simulink library "uas_pilot_model_r6"  (R2018b)
settings: Solver=VariableStepAuto  StartTime=0.0  StopTime=10.0  RelTol=1e-3
values from neighbouring files (symbols this model uses):
  deterministicMode = false    [HeuristicOperatorModelR6.m]
undefined symbols (not defined in the file or in its folder): alt_k, alt_offset, alt_theta, coord_delay_k, coord_delay_min, coord_delay_theta, dt, max_hdg_diff, mean_exec_delay, mean_initial_delay, mean_upd_times, min_exec_delay, min_initial_delay, min_upd_times, operator_enabled, prob_descend, prob_follow_min, prob_turn, prob_turn_left, rng_seed_coord, rng_seed_execution, rng_seed_horz, rng_seed_horz_vs_vert, rng_seed_initial, rng_seed_update, rng_seed_vert, turn_k, turn_k_alt, turn_offset, turn_offset_alt, turn_theta, turn_theta_alt
libraries: simulink x10
(part 1 of 2)
settings Model: Creator=RA24876  LastModifiedBy=PE29732
settings SFSimCC: SimUseLocalCustomCode=off
settings RTWCC: RTWUseLocalCustomCode=off
settings CodeAppCC: StateflowObjectComments=on

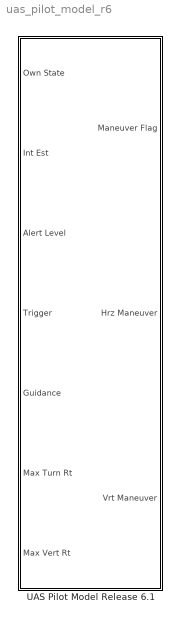
== system uas_pilot_model_r6 ==
  UAS Pilot Model Release 6.1 : Subsystem  TreatAsAtomicUnit=on  mask{dt=dt, operator_enabled=operator_enabled, deterministicMode=deterministicMode, mean_initial_delay=mean_initial_delay, min_initial_delay=min_initial_delay, coord_delay_k=coord_delay_k, coord_delay_theta=coord_delay_theta, coord_delay_min=coord_delay_min, mean_exec_delay=mean_exec_delay, min_exec_delay=min_exec_delay, min_upd_times=min_upd_times, mean_upd_times=mean_upd_times, rng_seed_initial=rng_seed_initial, rng_seed_coord=rng_seed_coord, rng_seed_execution=rng_seed_execution, rng_seed_update=rng_seed_update, prob_follow_min=prob_follow_min, prob_turn_left=prob_turn_left, prob_turn_table=prob_turn, max_hdg_diff=max_hdg_diff, prob_descend=prob_descend, turn_k=turn_k, turn_theta=turn_theta, turn_offset=turn_offset, turn_k_alt=turn_k_alt, turn_theta_alt=turn_theta_alt, turn_offset_alt=turn_offset_alt, alt_k=alt_k, alt_theta=alt_theta, alt_offset=alt_offset, rng_seed_horz=rng_seed_horz, rng_seed_vert=rng_seed_vert, rng_seed_horz_vs_vert=rng_seed_horz_vs_vert, mental_filter_samples=0, mental_filter_climb_thresh=0, mental_filter_turn_thresh=0}
      mask prompts: dt "Sample Time (s)"; operator_enabled "Enable Pilot Model (T/F)"; deterministicMode "Deterministic Mode"; mean_initial_delay "Mean Initial Delay (s)"; min_initial_delay "Minimum Initial Delay (s)"; coord_delay_k "Coordination Delay Gamma Distribution Shape Parameter, k"; coord_delay_theta "Coordination Delay Gamma Distribuition Scale Parameter, theta"; coord_delay_min "Minimum Coordination Delay (s)"; mean_exec_delay "Mean Execution Delay (s)"; min_exec_delay "Minimum Execution Delay (s)"; min_upd_times "Minimum Maneuve Update Times by Alert Level (s)"; mean_upd_times "Mean Maneuver Update Time by Alert Level (s)"; rng_seed_initial "Random Seed (Initial Delay)"; rng_seed_coord "Random Seed (Coord Delay)"; rng_seed_execution "Random Seed (Exec Delay)"; rng_seed_update "Random Seed (Update Delay)"; prob_follow_min "Probability of Following Minimum Guidance"; prob_turn_left "Probability of Turning Left"; prob_turn_table "Probability of Choosing Turn"; max_hdg_diff "Maximum Heading Difference to Override (deg)"; prob_descend "Probability of Descend vs. Climb"; turn_k "Primary Turn Magnitude Gamma Distribution Shape Parameter"; turn_theta "Primary Turn Magnitude Gamma Distribution Scale Parameter"; turn_offset "Primary Turn Magnitude Offset (deg)"; turn_k_alt "Alternate Turn Magnitude Shape Parameter"; turn_theta_alt "Alternate Turn Magnitude Scale Parameter"; turn_offset_alt "Alternate Turn Magnitude Offset"; alt_k "Altitude Gamma Distribution Shape Parameter"; alt_theta "Altitude Gamma Distribution Scale Parameter"; alt_offset "Altitude Offset (ft)"; rng_seed_horz "Random Seed (Horz Maneuver)"; rng_seed_vert "Random Seed (Vert Maneuver)"; rng_seed_horz_vs_vert "Random Seed (Turn vs. Climb)"; mental_filter_samples "Number of Samples for Mental Filter"; mental_filter_climb_thresh "Mental Filter Climb Threshold (fps)"; mental_filter_turn_thresh "Mental Filter Turn Threshold (rad)"
      mask DialogControl DescGroupVar Prompt: UAS Pilot Model
      mask DialogControl DescTextVar Prompt: Response of UAS pilot to intruder causing a DAA alert

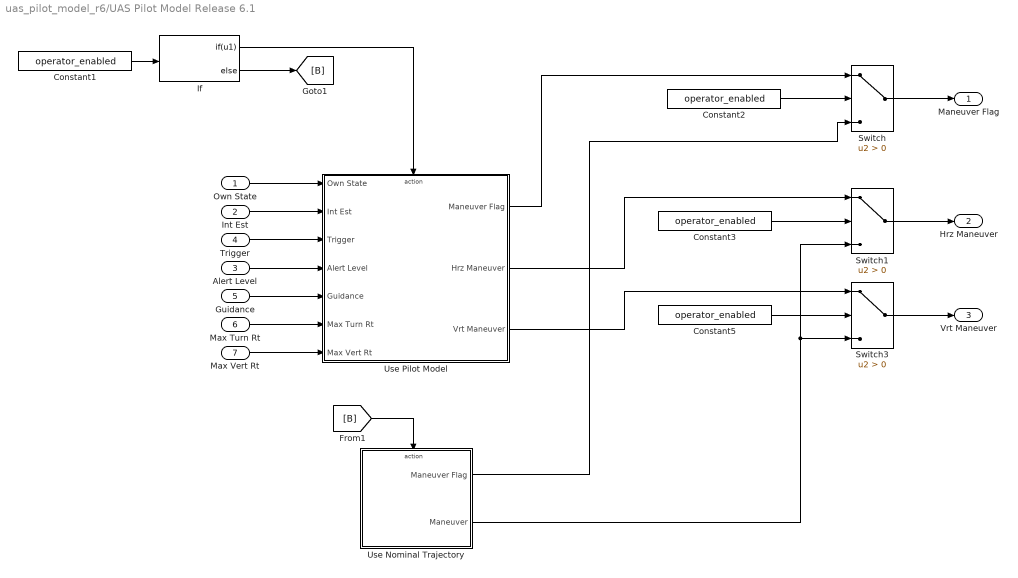
== system uas_pilot_model_r6/UAS Pilot Model Release 6.1 ==
  Own State : Inport  OutDataTypeStr=Bus: AircraftState
  Int Est : Inport  Port=2  OutDataTypeStr=Bus: AircraftEstimate
  Alert Level : Inport  Port=3
  Trigger : Inport  Port=4
  Guidance : Inport  Port=5
  Max Turn Rt : Inport  Port=6
  Max Vert Rt : Inport  Port=7
  Constant{1..3,5} (4 alike) : Constant  Value=operator_enabled  SampleTime=1
  If : If  IfExpression=u1
  Switch : Switch  Criteria=u2 > Threshold
  Switch1 : Switch  Criteria=u2 > Threshold
  Switch3 : Switch  Criteria=u2 > Threshold
  Use Nominal Trajectory : Subsystem  TreatAsAtomicUnit=on
  Use Pilot Model : Subsystem
  Maneuver Flag : Outport  OutDataTypeStr=boolean
  Hrz Maneuver : Outport  Port=2
  Vrt Maneuver : Outport  Port=3
  wires:
  Constant1/1 -> If/1
  If/2 -> [B]
  [B] -> Use Nominal Trajectory/Action
  Own State/1 -> Use Pilot Model/1(Own State)
  Int Est/1 -> Use Pilot Model/2(Int Est)
  If/1 -> Use Pilot Model/Action
  Switch/1 -> Maneuver Flag/1
  Constant2/1 -> Switch/2
  Use Pilot Model/1(Maneuver Flag) -> Switch/1
  Constant3/1 -> Switch1/2
  Use Pilot Model/2(Hrz Maneuver) -> Switch1/1
  Use Nominal Trajectory/1(Maneuver Flag) -> Switch/3
  Guidance/1 -> Use Pilot Model/5(Guidance)
  Constant5/1 -> Switch3/2
  Use Pilot Model/3(Vrt Maneuver) -> Switch3/1
  Use Nominal Trajectory/2(Maneuver) -> Switch3/3, Switch1/3
  Switch1/1 -> Hrz Maneuver/1
  Switch3/1 -> Vrt Maneuver/1
  Trigger/1 -> Use Pilot Model/3(Trigger)
  Alert Level/1 -> Use Pilot Model/4(Alert Level)
  Max Turn Rt/1 -> Use Pilot Model/6(Max Turn Rt)
  Max Vert Rt/1 -> Use Pilot Model/7(Max Vert Rt)

== system uas_pilot_model_r6/UAS Pilot Model Release 6.1/Use Nominal Trajectory ==
  Action Port : ActionPort
  Constant : Constant  Value=false
  Null Maneuver : Subsystem
  Maneuver Flag : Outport  InitialOutput=0
  Maneuver : Outport  Port=2  InitialOutput=0
  wires:
  Null Maneuver/1(Null) -> Maneuver/1
  Constant/1 -> Maneuver Flag/1

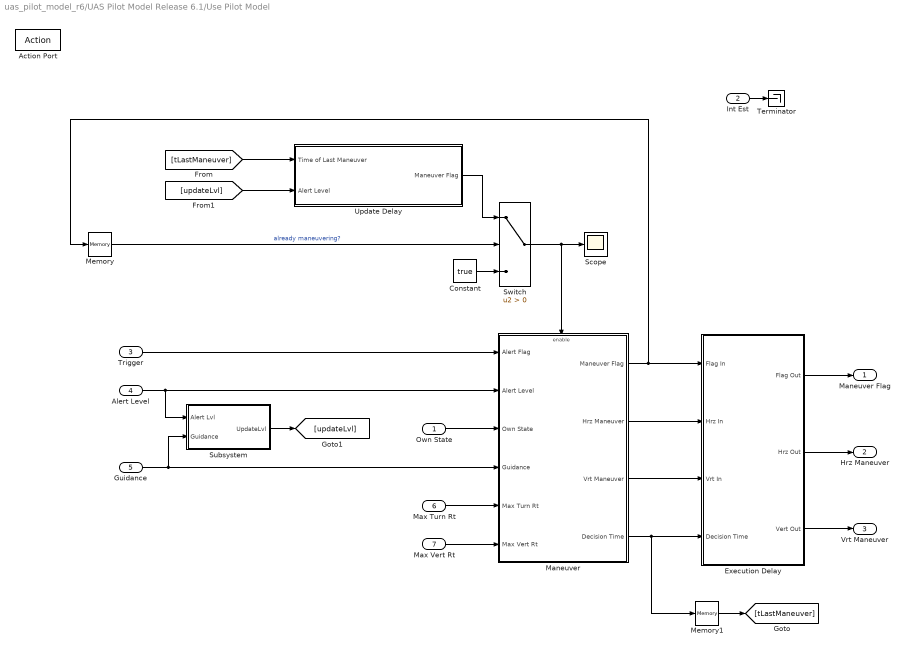
== system uas_pilot_model_r6/UAS Pilot Model Release 6.1/Use Pilot Model ==
  Own State : Inport  OutDataTypeStr=Bus: AircraftState
  Int Est : Inport  Port=2  OutDataTypeStr=Bus: AircraftEstimate
  Trigger : Inport  Port=3
  Alert Level : Inport  Port=4
  Guidance : Inport  Port=5
  Max Turn Rt : Inport  Port=6
  Max Vert Rt : Inport  Port=7
  Action Port : ActionPort
  Constant : Constant  Value=true
  Execution Delay : Subsystem
  Maneuver : Subsystem
  Memory : Memory  InheritSampleTime=on
  Memory1 : Memory  InheritSampleTime=on
  Scope : Scope
  Subsystem : Subsystem
  Switch : Switch  Criteria=u2 > Threshold
  Terminator : Terminator
  Update Delay : Subsystem
  Maneuver Flag : Outport  OutDataTypeStr=boolean
  Hrz Maneuver : Outport  Port=2
  Vrt Maneuver : Outport  Port=3
  wires:
  Maneuver/1(Maneuver Flag) -> Execution Delay/1(Flag In), Memory/1
  Guidance/1 -> Subsystem/2(Guidance), Maneuver/4(Guidance)
  Int Est/1 -> Terminator/1
  Constant/1 -> Switch/3
  Memory/1 -> Switch/2  "already maneuvering?"
  Own State/1 -> Maneuver/3(Own State)
  Trigger/1 -> Maneuver/1(Alert Flag)
  Alert Level/1 -> Subsystem/1(Alert Lvl), Maneuver/2(Alert Level)
  Switch/1 -> Maneuver/Enable, Scope/1
  Maneuver/2(Hrz Maneuver) -> Execution Delay/2(Hrz In)
  Maneuver/3(Vrt Maneuver) -> Execution Delay/3(Vrt In)
  Update Delay/1(Maneuver Flag) -> Switch/1
  Maneuver/4(Decision Time) -> Memory1/1, Execution Delay/4(Decision Time)
  Memory1/1 -> [tLastManeuver]
  [tLastManeuver] -> Update Delay/1(Time of Last Maneuver)
  Subsystem/1(UpdateLvl) -> [updateLvl]
  [updateLvl] -> Update Delay/2(Alert Level)
  Max Turn Rt/1 -> Maneuver/5(Max Turn Rt)
  Max Vert Rt/1 -> Maneuver/6(Max Vert Rt)
  Execution Delay/1(Flag Out) -> Maneuver Flag/1
  Execution Delay/2(Hrz Out) -> Hrz Maneuver/1
  Execution Delay/3(Vert Out) -> Vrt Maneuver/1

== system uas_pilot_model_r6/UAS Pilot Model Release 6.1/Use Nominal Trajectory/Null Maneuver ==
  Bus Creator : BusCreator  Inputs=5  OutDataTypeStr=Bus: AvoidanceManeuver
  Constant{,1..3} (4 alike) : Constant  Value=0
  Digital Clock : DigitalClock  SampleTime=dt
  Null : Outport
  wires:
  Constant2/1 -> Bus Creator/5  "wc_flag"
  Constant/1 -> Bus Creator/2  "type"
  Constant1/1 -> Bus Creator/3  "desired_state"
  Digital Clock/1 -> Bus Creator/1  "time"
  Bus Creator/1 -> Null/1
  Constant3/1 -> Bus Creator/4  "reference_state"

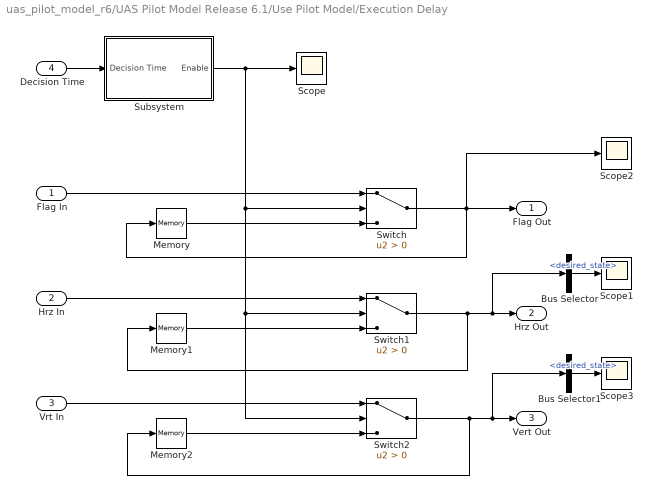
== system uas_pilot_model_r6/UAS Pilot Model Release 6.1/Use Pilot Model/Execution Delay ==
  Flag In : Inport
  Hrz In : Inport  Port=2
  Vrt In : Inport  Port=3
  Decision Time : Inport  Port=4
  Bus Selector : BusSelector  OutputSignals=desired_state
  Bus Selector1 : BusSelector  OutputSignals=desired_state
  Memory : Memory  InheritSampleTime=on
  Memory1 : Memory  InheritSampleTime=on
  Memory2 : Memory  InheritSampleTime=on
  Scope{,1..3} (4 alike) : Scope
  Subsystem : Subsystem
  Switch : Switch  Criteria=u2 > Threshold
  Switch1 : Switch  Criteria=u2 > Threshold
  Switch2 : Switch  Criteria=u2 > Threshold
  Flag Out : Outport
  Hrz Out : Outport  Port=2
  Vert Out : Outport  Port=3
  wires:
  Switch/1 -> Scope2/1, Memory/1, Flag Out/1
  Switch1/1 -> Memory1/1, Bus Selector/1, Hrz Out/1
  Flag In/1 -> Switch/1
  Vrt In/1 -> Switch2/1
  Hrz In/1 -> Switch1/1
  Memory/1 -> Switch/3
  Memory1/1 -> Switch1/3
  Memory2/1 -> Switch2/3
  Subsystem/1(Enable) -> Scope/1, Switch/2, Switch1/2, Switch2/2
  Decision Time/1 -> Subsystem/1(Decision Time)
  Bus Selector/1 -> Scope1/1  "<desired_state>"
  Switch2/1 -> Memory2/1, Bus Selector1/1, Vert Out/1
  Bus Selector1/1 -> Scope3/1  "<desired_state>"

== system uas_pilot_model_r6/UAS Pilot Model Release 6.1/Use Pilot Model/Maneuver ==
  Alert Flag : Inport
  Alert Level : Inport  Port=2
  Own State : Inport  Port=3
  Guidance : Inport  Port=4
  Max Turn Rt : Inport  Port=5
  Max Vert Rt : Inport  Port=6
  Enable : EnablePort
  Coordination Delay : Subsystem
  Initial Delay : Subsystem
  Logical Operator : Logic  Operator=OR  AllPortsSameDT=off  OutDataTypeStr=boolean
  Maneuver Selection : Subsystem  TreatAsAtomicUnit=on
  Memory : Memory  InheritSampleTime=on
  Scope1 : Scope
  Maneuver Flag : Outport
  Hrz Maneuver : Outport  Port=2
  Vrt Maneuver : Outport  Port=3
  Decision Time : Outport  Port=4
  wires:
  Guidance/1 -> Maneuver Selection/2(Guidance)
  Memory/1 -> Coordination Delay/1(Maneuver Flag), Logical Operator/1, Initial Delay/1(Maneuver Flag)
  Initial Delay/1(Flag Out) -> Coordination Delay/2(Flag In)
  Alert Level/1 -> Coordination Delay/4(Alert Level)
  Coordination Delay/1(Flag Out) -> Scope1/1, Maneuver Selection/Enable
  Own State/1 -> Maneuver Selection/1(Own State)
  Alert Flag/1 -> Logical Operator/2
  Logical Operator/1 -> Coordination Delay/3(Alert Flag), Initial Delay/2(Alert Flag)
  Max Turn Rt/1 -> Maneuver Selection/3(Max Turn Rt)
  Max Vert Rt/1 -> Maneuver Selection/4(Max Vert Rt)
  Maneuver Selection/4(Decision Time) -> Decision Time/1
  Maneuver Selection/3(Vrt Maneuver) -> Vrt Maneuver/1
  Maneuver Selection/2(Hrz Maneuver) -> Hrz Maneuver/1
  Maneuver Selection/1(Maneuver Flag) -> Maneuver Flag/1, Memory/1

== system uas_pilot_model_r6/UAS Pilot Model Release 6.1/Use Pilot Model/Subsystem ==
  note: Pass through current alert level unless any recovery guidance is present, in which case set alert level to 5
  note: See if horizontal guidance includes any recovery bands (value =1)
  note: Alert Levels:
      | 0 = no alert
      | 1 = proximate alert
      | 2 = preventive alert
      | 3 = corrective alert
      | 4 = warning alert
      | 5 = recovery bands or WCV
  Alert Lvl : Inport
  Guidance : Inport  Port=2
  Compare To Constant : simulink/Logic and Bit Operations/Compare To Constant  relop===  const=1  OutDataTypeStr=boolean
  Compare To Zero : simulink/Logic and Bit Operations/Compare To Zero  relop=>  OutDataTypeStr=boolean
  Constant : Constant  Value=5
  Selector : Selector  InputPortWidth=283  IndexOptions=Index vector (dialog)  Indices=[1:271]  OutputSizes=1
  Sum of Elements : Sum  Inputs=+
  Switch1 : Switch  Criteria=u2 > Threshold
  UpdateLvl : Outport
  wires:
  Switch1/1 -> UpdateLvl/1
  Compare To Zero/1 -> Switch1/2
  Constant/1 -> Switch1/1
  Alert Lvl/1 -> Switch1/3
  Guidance/1 -> Selector/1
  Compare To Constant/1 -> Sum of Elements/1
  Sum of Elements/1 -> Compare To Zero/1
  Selector/1 -> Compare To Constant/1

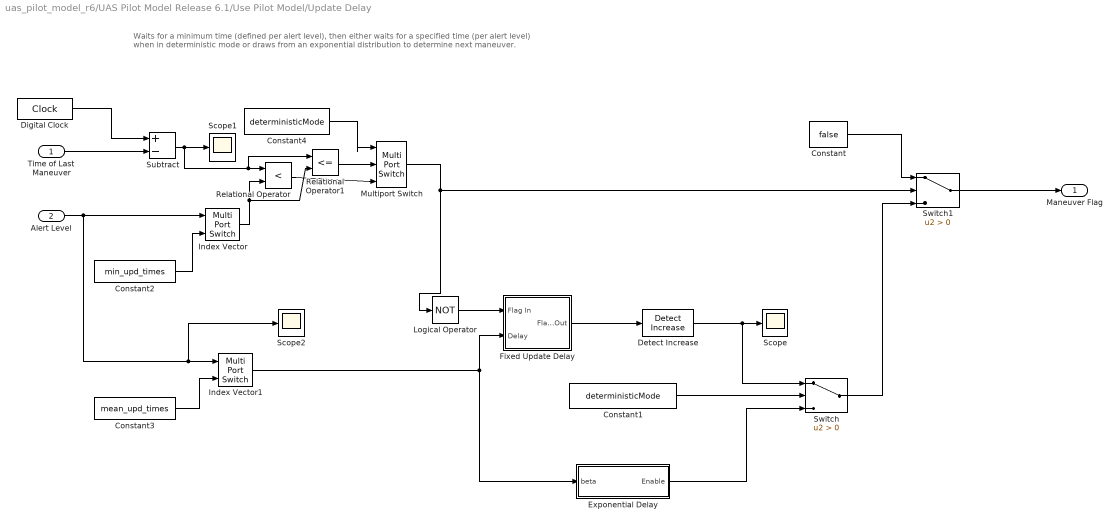
== system uas_pilot_model_r6/UAS Pilot Model Release 6.1/Use Pilot Model/Update Delay ==
  note: Waits for a minimum time (defined per alert level), then either waits for a specified time (per alert level)
      | when in deterministic mode or draws from an exponential distribution to determine next maneuver.
  Time of Last Maneuver : Inport
  Alert Level : Inport  Port=2
  Constant : Constant  Value=false
  Constant1 : Constant  Value=deterministicMode
  Constant2 : Constant  Value=min_upd_times
  Constant3 : Constant  Value=mean_upd_times
  Constant4 : Constant  Value=deterministicMode
  Detect Increase : simulink/Logic and Bit Operations/Detect Increase  vinit=0.0  OutDataTypeStr=boolean
  Digital Clock : DigitalClock
  Exponential Delay : Subsystem  mask(Exponentially-Distributed Delay){dt=dt, seed=rng_seed_update}
      mask prompts: dt "Sample time (seconds):"; seed "Random seed:"
      mask help:
      | Outputs whether a delay follows an exponential distribution with the specified mean time has completed.
      |
      | Because the exponential distribution is memoryless, the probability of finishing the delay at the current timestep is independent of previous timesteps.
  Fixed Update Delay : Subsystem
  Index Vector : MultiPortSwitch  DataPortOrder=Zero-based contiguous  Inputs=1  zeroidx=on
  Index Vector1 : MultiPortSwitch  DataPortOrder=Zero-based contiguous  Inputs=1  zeroidx=on
  Logical Operator : Logic  Operator=NOT  AllPortsSameDT=off  OutDataTypeStr=boolean
  Multiport Switch : MultiPortSwitch  DataPortOrder=Specify indices  Inputs={1, 0}  DataPortIndices={1, 0}
  Relational Operator : RelationalOperator  Operator=<  OutDataTypeStr=boolean  RndMeth=Nearest
  Relational Operator1 : RelationalOperator  Operator=<=  OutDataTypeStr=boolean  RndMeth=Nearest
  Scope : Scope
  Scope1 : Scope
  Scope2 : Scope
  Subtract : Sum  Inputs=+-
  Switch : Switch  Criteria=u2 > Threshold
  Switch1 : Switch  Criteria=u2 > Threshold
  Maneuver Flag : Outport
  wires:
  Switch1/1 -> Maneuver Flag/1
  Constant1/1 -> Switch/2
  Exponential Delay/1(Enable) -> Switch/3
  Multiport Switch/1 -> Switch1/2, Logical Operator/1
  Fixed Update Delay/1(Flag Out) -> Detect Increase/1
  Detect Increase/1 -> Scope/1, Switch/1
  Alert Level/1 -> Index Vector1/1, Scope2/1, Index Vector/1
  Constant2/1 -> Index Vector/2
  Constant3/1 -> Index Vector1/2
  Index Vector/1 -> Relational Operator1/2, Relational Operator/2
  Constant/1 -> Switch1/1
  Index Vector1/1 -> Exponential Delay/1(beta), Fixed Update Delay/2(Delay)
  Logical Operator/1 -> Fixed Update Delay/1(Flag In)
  Switch/1 -> Switch1/3
  Time of Last Maneuver/1 -> Subtract/2
  Digital Clock/1 -> Subtract/1
  Subtract/1 -> Scope1/1, Relational Operator1/1, Relational Operator/1
  Relational Operator/1 -> Multiport Switch/3
  Relational Operator1/1 -> Multiport Switch/2
  Constant4/1 -> Multiport Switch/1

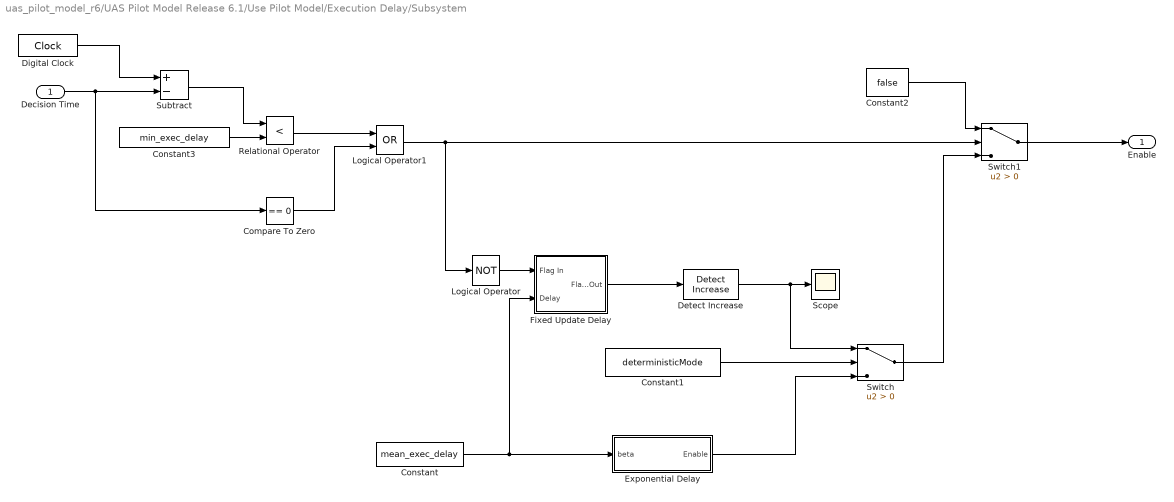
== system uas_pilot_model_r6/UAS Pilot Model Release 6.1/Use Pilot Model/Execution Delay/Subsystem ==
  Decision Time : Inport
  Compare To Zero : simulink/Logic and Bit Operations/Compare To Zero  relop===  OutDataTypeStr=boolean
  Constant : Constant  Value=mean_exec_delay
  Constant1 : Constant  Value=deterministicMode
  Constant2 : Constant  Value=false
  Constant3 : Constant  Value=min_exec_delay
  Detect Increase : simulink/Logic and Bit Operations/Detect Increase  vinit=0.0  InputProcessing=Inherited  OutDataTypeStr=boolean
  Digital Clock : DigitalClock
  Exponential Delay : Subsystem  mask(Exponentially-Distributed Delay){dt=dt, seed=rng_seed_execution}
      mask prompts: dt "Sample time (seconds):"; seed "Random seed:"
      mask help:
      | Outputs whether a delay follows an exponential distribution with the specified mean time has completed.
      |
      | Because the exponential distribution is memoryless, the probability of finishing the delay at the current timestep is independent of previous timesteps.
  Fixed Update Delay : Subsystem
  Logical Operator : Logic  Operator=NOT  AllPortsSameDT=off  OutDataTypeStr=boolean
  Logical Operator1 : Logic  Operator=OR  AllPortsSameDT=off  OutDataTypeStr=boolean
  Relational Operator : RelationalOperator  Operator=<  OutDataTypeStr=boolean  RndMeth=Nearest
  Scope : Scope
  Subtract : Sum  Inputs=+-
  Switch : Switch  Criteria=u2 > Threshold
  Switch1 : Switch  Criteria=u2 > Threshold
  Enable : Outport
  wires:
  Constant1/1 -> Switch/2
  Exponential Delay/1(Enable) -> Switch/3
  Fixed Update Delay/1(Flag Out) -> Detect Increase/1
  Detect Increase/1 -> Scope/1, Switch/1
  Constant/1 -> Exponential Delay/1(beta), Fixed Update Delay/2(Delay)
  Logical Operator/1 -> Fixed Update Delay/1(Flag In)
  Switch1/1 -> Enable/1
  Logical Operator1/1 -> Logical Operator/1, Switch1/2
  Constant3/1 -> Relational Operator/2
  Constant2/1 -> Switch1/1
  Decision Time/1 -> Compare To Zero/1, Subtract/2
  Digital Clock/1 -> Subtract/1
  Subtract/1 -> Relational Operator/1
  Switch/1 -> Switch1/3
  Relational Operator/1 -> Logical Operator1/1
  Compare To Zero/1 -> Logical Operator1/2

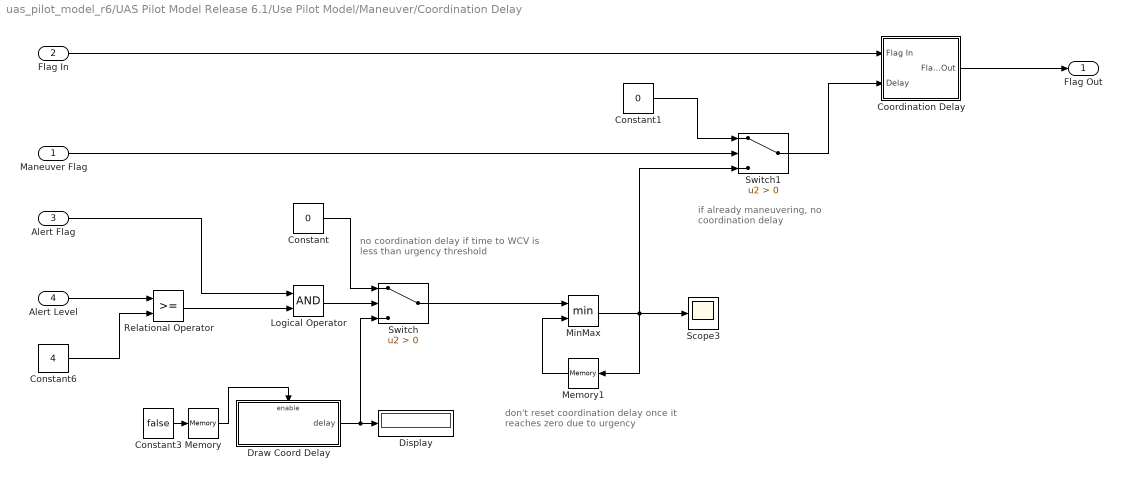
== system uas_pilot_model_r6/UAS Pilot Model Release 6.1/Use Pilot Model/Maneuver/Coordination Delay ==
  note: if already maneuvering, no
      | coordination delay
  note: no coordination delay if time to WCV
      | is less than urgency threshold
  note: don't reset coordination delay once
      | it reaches zero due to urgency
  Maneuver Flag : Inport
  Flag In : Inport  Port=2
  Alert Flag : Inport  Port=3
  Alert Level : Inport  Port=4
  Constant : Constant  Value=0
  Constant1 : Constant  Value=0
  Constant3 : Constant  Value=false
  Constant6 : Constant  Value=4
  Coordination Delay : Subsystem
  Display : Display
  Draw Coord Delay : Subsystem  TreatAsAtomicUnit=on  mask{k=coord_delay_k, theta=coord_delay_theta, offset=coord_delay_min, seed=rng_seed_coord}
      mask prompts: k "Gamma Distribution Shape Parameter, k"; theta "Gamma Distribution Scale Parameter, theta"
  Logical Operator : Logic  AllPortsSameDT=off  OutDataTypeStr=boolean
  Memory : Memory  InitialCondition=true  InheritSampleTime=on
  Memory1 : Memory  InitialCondition=1000  InheritSampleTime=on
  MinMax : MinMax  Inputs=2
  Relational Operator : RelationalOperator  OutDataTypeStr=boolean  RndMeth=Nearest
  Scope3 : Scope
  Switch : Switch  Criteria=u2 > Threshold
  Switch1 : Switch  Criteria=u2 > Threshold
  Flag Out : Outport
  wires:
  Alert Flag/1 -> Logical Operator/1
  Flag In/1 -> Coordination Delay/1(Flag In)
  Switch/1 -> MinMax/1
  Memory1/1 -> MinMax/2
  MinMax/1 -> Switch1/3, Scope3/1, Memory1/1
  Draw Coord Delay/1(delay) -> Display/1, Switch/3
  Logical Operator/1 -> Switch/2
  Constant6/1 -> Relational Operator/2
  Relational Operator/1 -> Logical Operator/2
  Coordination Delay/1(Flag Out) -> Flag Out/1
  Alert Level/1 -> Relational Operator/1
  Constant/1 -> Switch/1
  Switch1/1 -> Coordination Delay/2(Delay)
  Constant1/1 -> Switch1/1
  Maneuver Flag/1 -> Switch1/2
  Memory/1 -> Draw Coord Delay/Enable
  Constant3/1 -> Memory/1

== system uas_pilot_model_r6/UAS Pilot Model Release 6.1/Use Pilot Model/Maneuver/Initial Delay ==
  note: If already maneuvering, no delay
      | for subsequent maneuvers
  Maneuver Flag : Inport
  Alert Flag : Inport  Port=2
  Constant1 : Constant  Value=0
  Constant3 : Constant  Value=false
  Display : Display
  Draw Initial Delay : Subsystem  TreatAsAtomicUnit=on  mask{mu=mean_initial_delay, offset=min_initial_delay, seed=rng_seed_initial}
      mask prompts: mu "Exponential Distribution Mean Parameter, k"
  Memory : Memory  InitialCondition=true  InheritSampleTime=on
  Switch1 : Switch  Criteria=u2 > Threshold
  Wait for Intruder to Give Way : Subsystem
  Flag Out : Outport
  wires:
  Alert Flag/1 -> Wait for Intruder to Give Way/1(Flag In)
  Wait for Intruder to Give Way/1(Flag Out) -> Flag Out/1
  Maneuver Flag/1 -> Switch1/2
  Switch1/1 -> Wait for Intruder to Give Way/2(Delay)
  Draw Initial Delay/1(delay) -> Switch1/3, Display/1
  Constant1/1 -> Switch1/1
  Memory/1 -> Draw Initial Delay/Enable
  Constant3/1 -> Memory/1

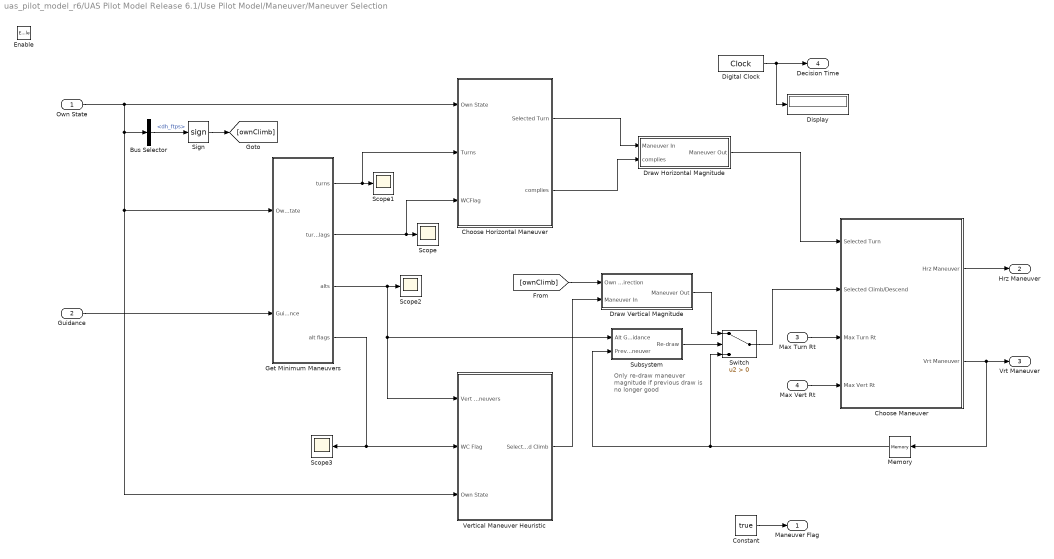
== system uas_pilot_model_r6/UAS Pilot Model Release 6.1/Use Pilot Model/Maneuver/Maneuver Selection ==
  note: Only re-draw maneuver
      | magnitude if previous
      | draw is no longer good
  Own State : Inport
  Guidance : Inport  Port=2
  Max Turn Rt : Inport  Port=3
  Max Vert Rt : Inport  Port=4
  Enable : EnablePort
  Bus Selector : BusSelector  OutputSignals=dh_ftps
  Choose Horizontal Maneuver : Subsystem
  Choose Maneuver : Subsystem
  Constant : Constant  Value=true
  Digital Clock : DigitalClock
  Display : Display
  Draw Horizontal Magnitude : Subsystem
  Draw Vertical Magnitude : Subsystem
  Get Minimum Maneuvers : Subsystem
  Memory : Memory  InheritSampleTime=on
  Scope{,1..3} (4 alike) : Scope
  Sign : Signum
  Subsystem : Subsystem
  Switch : Switch  Criteria=u2 > Threshold
  Vertical Maneuver Heuristic : Subsystem
  Maneuver Flag : Outport  InitialOutput=0
  Hrz Maneuver : Outport  Port=2  OutDataTypeStr=Bus: AvoidanceManeuver  InitialOutput=0
  Vrt Maneuver : Outport  Port=3  OutDataTypeStr=Bus: AvoidanceManeuver  InitialOutput=0
  Decision Time : Outport  Port=4
  wires:
  Switch/1 -> Choose Maneuver/2(Selected Climb/Descend)
  Subsystem/1(Re-draw) -> Switch/2
  Memory/1 -> Subsystem/2(Prev Maneuver), Switch/3
  Choose Horizontal Maneuver/2(complies) -> Draw Horizontal Magnitude/2(complies)
  Get Minimum Maneuvers/1(turns) -> Choose Horizontal Maneuver/2(Turns), Scope1/1
  Get Minimum Maneuvers/2(turn flags) -> Choose Horizontal Maneuver/3(WCFlag), Scope/1
  Get Minimum Maneuvers/3(alts) -> Vertical Maneuver Heuristic/1(Vert Maneuvers), Subsystem/1(Alt Guidance), Scope2/1
  Get Minimum Maneuvers/4(alt flags) -> Vertical Maneuver Heuristic/2(WC Flag), Scope3/1
  Digital Clock/1 -> Display/1, Decision Time/1
  Constant/1 -> Maneuver Flag/1
  Own State/1 -> Choose Horizontal Maneuver/1(Own State), Get Minimum Maneuvers/1(Own State), Vertical Maneuver Heuristic/3(Own State), Bus Selector/1
  Choose Maneuver/1(Hrz Maneuver) -> Hrz Maneuver/1
  Choose Horizontal Maneuver/1(Selected Turn) -> Draw Horizontal Magnitude/1(Maneuver In)
  Vertical Maneuver Heuristic/1(Selected Climb) -> Draw Vertical Magnitude/2(Maneuver In)
  Guidance/1 -> Get Minimum Maneuvers/2(Guidance)
  Choose Maneuver/2(Vrt Maneuver) -> Vrt Maneuver/1, Memory/1
  Draw Horizontal Magnitude/1(Maneuver Out) -> Choose Maneuver/1(Selected Turn)
  Draw Vertical Magnitude/1(Maneuver Out) -> Switch/1
  Max Turn Rt/1 -> Choose Maneuver/3(Max Turn Rt)
  Max Vert Rt/1 -> Choose Maneuver/4(Max Vert Rt)
  Bus Selector/1 -> Sign/1  "<dh_ftps>"
  Sign/1 -> [ownClimb]
  [ownClimb] -> Draw Vertical Magnitude/1(Own Vertical Direction)

== system uas_pilot_model_r6/UAS Pilot Model Release 6.1/Use Pilot Model/Update Delay/Exponential Delay ==
  note: Delay exponentially distributed with mean interarrival time of beta.
      | Delay over (returns true) if X <= 1-exp(-dt/beta) where X is uniformly distributed between 0 and 1.
  beta : Inport
  Constant : Constant
  Divide : Product  Inputs=*/
  Math Function : Math  SaturateOnIntegerOverflow=on
  Relational Operator : RelationalOperator  Operator=<=  OutDataTypeStr=boolean  RndMeth=Nearest
  Sample Time : Constant  Value=dt
  Subtract : Sum  Inputs=+-
  Unary Minus : UnaryMinus
  Uniform Random Number : UniformRandomNumber  Minimum=0  Seed=seed  SampleTime=dt
  Enable : Outport  OutDataTypeStr=boolean
  wires:
  beta/1 -> Divide/2
  Unary Minus/1 -> Divide/1
  Constant/1 -> Subtract/1
  Sample Time/1 -> Unary Minus/1
  Math Function/1 -> Subtract/2
  Subtract/1 -> Relational Operator/2
  Uniform Random Number/1 -> Relational Operator/1
  Divide/1 -> Math Function/1
  Relational Operator/1 -> Enable/1

== system uas_pilot_model_r6/UAS Pilot Model Release 6.1/Use Pilot Model/Update Delay/Fixed Update Delay ==
  Flag In : Inport
  Delay : Inport  Port=2
  Add : Sum
  Constant1 : Constant  Value=0
  Constant2 : Constant
  Memory : Memory  InheritSampleTime=on
  Relational Operator : RelationalOperator  Operator=>  OutDataTypeStr=boolean  RndMeth=Nearest
  Switch : Switch  Criteria=u2 > Threshold
  Flag Out : Outport
  wires:
  Add/1 -> Switch/1
  Constant2/1 -> Add/1
  Flag In/1 -> Switch/2
  Memory/1 -> Add/2
  Constant1/1 -> Switch/3
  Switch/1 -> Relational Operator/1, Memory/1
  Relational Operator/1 -> Flag Out/1
  Delay/1 -> Relational Operator/2

== system uas_pilot_model_r6/UAS Pilot Model Release 6.1/Use Pilot Model/Execution Delay/Subsystem/Exponential Delay ==
  note: Delay exponentially distributed with mean interarrival time of beta.
      | Delay over (returns true) if X <= 1-exp(-dt/beta) where X is uniformly distributed between 0 and 1.
  beta : Inport
  Constant : Constant
  Divide : Product  Inputs=*/
  Math Function : Math  SaturateOnIntegerOverflow=on
  Relational Operator : RelationalOperator  Operator=<=  OutDataTypeStr=boolean  RndMeth=Nearest
  Sample Time : Constant  Value=dt
  Subtract : Sum  Inputs=+-
  Unary Minus : UnaryMinus
  Uniform Random Number : UniformRandomNumber  Minimum=0  Seed=seed  SampleTime=dt
  Enable : Outport  OutDataTypeStr=boolean
  wires:
  beta/1 -> Divide/2
  Unary Minus/1 -> Divide/1
  Constant/1 -> Subtract/1
  Sample Time/1 -> Unary Minus/1
  Math Function/1 -> Subtract/2
  Subtract/1 -> Relational Operator/2
  Uniform Random Number/1 -> Relational Operator/1
  Divide/1 -> Math Function/1
  Relational Operator/1 -> Enable/1

== system uas_pilot_model_r6/UAS Pilot Model Release 6.1/Use Pilot Model/Execution Delay/Subsystem/Fixed Update Delay ==
  Flag In : Inport
  Delay : Inport  Port=2
  Add : Sum
  Constant1 : Constant  Value=0
  Constant2 : Constant
  Memory : Memory  InheritSampleTime=on
  Relational Operator : RelationalOperator  Operator=>  OutDataTypeStr=boolean  RndMeth=Nearest
  Switch : Switch  Criteria=u2 > Threshold
  Flag Out : Outport
  wires:
  Add/1 -> Switch/1
  Constant2/1 -> Add/1
  Flag In/1 -> Switch/2
  Memory/1 -> Add/2
  Constant1/1 -> Switch/3
  Switch/1 -> Relational Operator/1, Memory/1
  Relational Operator/1 -> Flag Out/1
  Delay/1 -> Relational Operator/2

== system uas_pilot_model_r6/UAS Pilot Model Release 6.1/Use Pilot Model/Maneuver/Coordination Delay/Coordination Delay ==
  Flag In : Inport
  Delay : Inport  Port=2
  Add : Sum
  Constant1 : Constant  Value=0
  Constant2 : Constant
  Memory : Memory  InheritSampleTime=on
  Relational Operator : RelationalOperator  Operator=>  OutDataTypeStr=boolean  RndMeth=Nearest
  Switch : Switch  Criteria=u2 > Threshold
  Flag Out : Outport
  wires:
  Add/1 -> Switch/1
  Constant2/1 -> Add/1
  Flag In/1 -> Switch/2
  Memory/1 -> Add/2
  Constant1/1 -> Switch/3
  Switch/1 -> Relational Operator/1, Memory/1
  Relational Operator/1 -> Flag Out/1
  Delay/1 -> Relational Operator/2

== system uas_pilot_model_r6/UAS Pilot Model Release 6.1/Use Pilot Model/Maneuver/Coordination Delay/Draw Coord Delay ==
  Enable : EnablePort
  Generate Random Gamma Deviate : Subsystem  mask{k=k, theta=theta, offset=offset, seed=seed}
      mask prompts: k "Shape Parameter, k"; theta "Scale Parameter, theta"
  Rounding Function : Rounding  Operator=round
  delay : Outport  InitialOutput=0
  wires:
  Rounding Function/1 -> delay/1
  Generate Random Gamma Deviate/1(y) -> Rounding Function/1

== system uas_pilot_model_r6/UAS Pilot Model Release 6.1/Use Pilot Model/Maneuver/Initial Delay/Draw Initial Delay ==
  Enable : EnablePort
  Generate Random Exponential Deviate : Subsystem  mask{mu=mu, offset=offset, seed=seed}
      mask prompts: mu "Mean Parameter, mu"
  Rounding Function : Rounding  Operator=round
  delay : Outport  InitialOutput=0
  wires:
  Generate Random Exponential Deviate/1(y) -> Rounding Function/1
  Rounding Function/1 -> delay/1

== system uas_pilot_model_r6/UAS Pilot Model Release 6.1/Use Pilot Model/Maneuver/Initial Delay/Wait for Intruder to Give Way ==
  Flag In : Inport
  Delay : Inport  Port=2
  Add : Sum
  Constant1 : Constant  Value=0
  Constant2 : Constant
  Memory : Memory  InheritSampleTime=on
  Relational Operator : RelationalOperator  Operator=>  OutDataTypeStr=boolean  RndMeth=Nearest
  Switch : Switch  Criteria=u2 > Threshold
  Flag Out : Outport
  wires:
  Add/1 -> Switch/1
  Constant2/1 -> Add/1
  Flag In/1 -> Switch/2
  Memory/1 -> Add/2
  Constant1/1 -> Switch/3
  Switch/1 -> Relational Operator/1, Memory/1
  Relational Operator/1 -> Flag Out/1
  Delay/1 -> Relational Operator/2

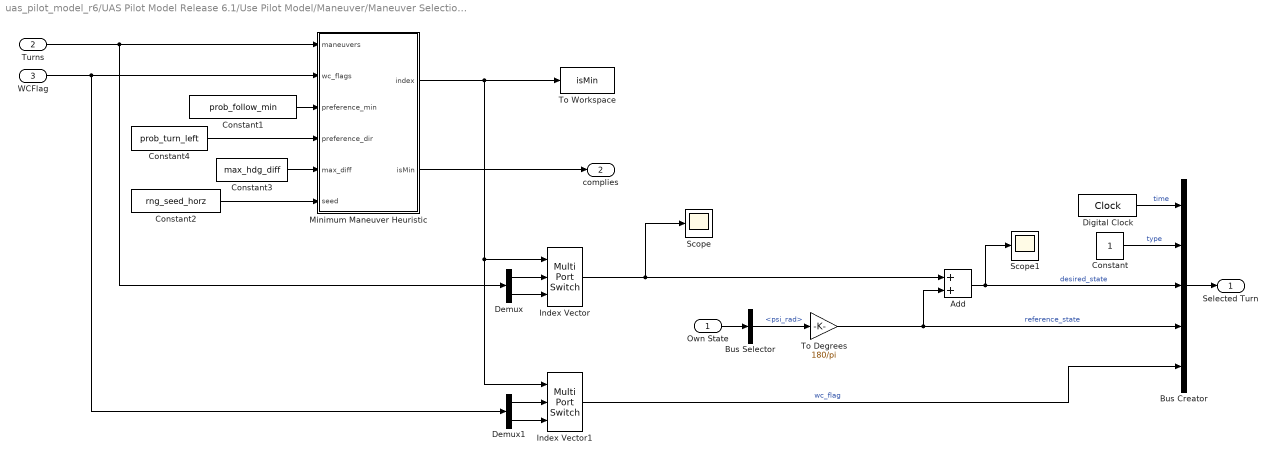
== system uas_pilot_model_r6/UAS Pilot Model Release 6.1/Use Pilot Model/Maneuver/Maneuver Selection/Choose Horizontal Maneuver ==
  Own State : Inport
  Turns : Inport  Port=2
  WCFlag : Inport  Port=3
  Add : Sum
  Bus Selector : BusSelector  OutputSignals=psi_rad
  Bus Creator : BusCreator  Inputs=5  OutDataTypeStr=Bus: AvoidanceManeuver
  Constant : Constant
  Constant1 : Constant  Value=prob_follow_min
  Constant2 : Constant  Value=rng_seed_horz
  Constant3 : Constant  Value=max_hdg_diff
  Constant4 : Constant  Value=prob_turn_left
  Demux : Demux  Outputs=2
  Demux1 : Demux  Outputs=2
  Digital Clock : DigitalClock  SampleTime=dt
  Index Vector : MultiPortSwitch  DataPortOrder=Specify indices  Inputs=2  DataPortIndices={1,2}
  Index Vector1 : MultiPortSwitch  DataPortOrder=Specify indices  Inputs=2  DataPortIndices={1,2}
  Minimum Maneuver Heuristic : MATLAB Function  TreatAsAtomicUnit=on
  Scope : Scope
  Scope1 : Scope
  To Degrees : Gain  Gain=180/pi
  To Workspace : ToWorkspace  VariableName=isMin  SaveFormat=Timeseries  SampleTime=-1
  Selected Turn : Outport  OutDataTypeStr=Bus: AvoidanceManeuver
  complies : Outport  Port=2  OutDataTypeStr=boolean
  wires:
  Minimum Maneuver Heuristic/2(isMin) -> complies/1
  WCFlag/1 -> Minimum Maneuver Heuristic/2(wc_flags), Demux1/1
  Turns/1 -> Minimum Maneuver Heuristic/1(maneuvers), Demux/1
  Bus Creator/1 -> Selected Turn/1
  Digital Clock/1 -> Bus Creator/1  "time"
  Index Vector1/1 -> Bus Creator/5  "wc_flag"
  Index Vector/1 -> Scope/1, Add/1
  Constant/1 -> Bus Creator/2  "type"
  Own State/1 -> Bus Selector/1
  Bus Selector/1 -> To Degrees/1  "<psi_rad>"
  Constant1/1 -> Minimum Maneuver Heuristic/3(preference_min)
  Constant2/1 -> Minimum Maneuver Heuristic/6(seed)
  Minimum Maneuver Heuristic/1(index) -> To Workspace/1, Index Vector1/1, Index Vector/1
  Demux/1 -> Index Vector/2
  Demux/2 -> Index Vector/3
  Demux1/1 -> Index Vector1/2
  Demux1/2 -> Index Vector1/3
  Constant3/1 -> Minimum Maneuver Heuristic/5(max_diff)
  Constant4/1 -> Minimum Maneuver Heuristic/4(preference_dir)
  To Degrees/1 -> Bus Creator/4, Add/2  "reference_state"
  Add/1 -> Bus Creator/3, Scope1/1  "desired_state"

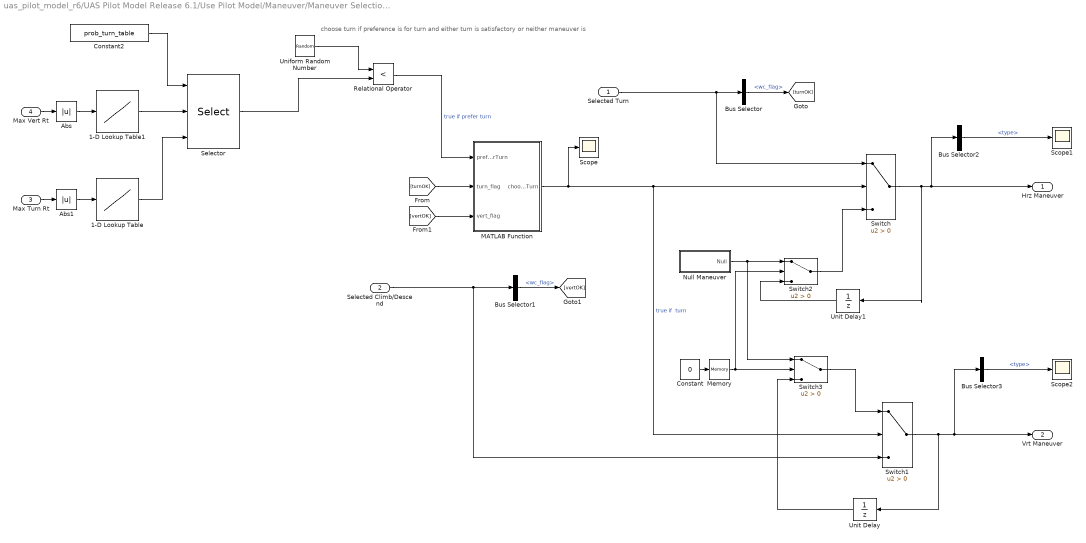
== system uas_pilot_model_r6/UAS Pilot Model Release 6.1/Use Pilot Model/Maneuver/Maneuver Selection/Choose Maneuver ==
  note: choose turn if preference is for turn and either turn is satisfactory or neither maneuver is
  Selected Turn : Inport
  Selected Climb/Descend : Inport  Port=2
  Max Turn Rt : Inport  Port=3
  Max Vert Rt : Inport  Port=4
  1-D Lookup Table : Lookup_n-D  NumberOfTableDimensions=1  BreakpointsForDimension1=[-1,0+1e-6,2+1e-6]  Table=[1,2,3]  InterpMethod=Flat  InternalRulePriority=Speed  RndMeth=Simplest  InputSameDT=on
  1-D Lookup Table1 : Lookup_n-D  NumberOfTableDimensions=1  BreakpointsForDimension1=[-1,0+1e-6,1000+1e-6]  Table=[1,2,3]  InterpMethod=Flat  InternalRulePriority=Speed  RndMeth=Simplest  InputSameDT=on
  Abs : Abs
  Abs1 : Abs
  Bus Selector2 : BusSelector  OutputSignals=type
  Bus Selector3 : BusSelector  OutputSignals=type
  Bus Selector : BusSelector  OutputSignals=wc_flag
  Bus Selector1 : BusSelector  OutputSignals=wc_flag
  Constant : Constant  Value=0
  Constant2 : Constant  Value=prob_turn_table
  MATLAB Function : MATLAB Function  TreatAsAtomicUnit=on
  Memory : Memory  InitialCondition=1  InheritSampleTime=on
  Null Maneuver : Subsystem
  Relational Operator : RelationalOperator  Operator=<  OutDataTypeStr=boolean  RndMeth=Nearest
  Scope : Scope
  Scope1 : Scope
  Scope2 : Scope
  Selector : Selector  NumberOfDimensions=2  InputPortWidth=3  IndexOptions=Index vector (port),Index vector (port)  Indices=[1 3],1  OutputSizes=1,1
  Switch{,1..3} (4 alike) : Switch  Criteria=u2 > Threshold
  Uniform Random Number : UniformRandomNumber  Minimum=0  Seed=rng_seed_horz_vs_vert  SampleTime=1
  Unit Delay : UnitDelay  SampleTime=-1
  Unit Delay1 : UnitDelay  SampleTime=-1
  Hrz Maneuver : Outport
  Vrt Maneuver : Outport  Port=2
  wires:
  Selected Climb/Descend/1 -> Switch1/3, Bus Selector1/1
  Selected Turn/1 -> Switch/1, Bus Selector/1
  Uniform Random Number/1 -> Relational Operator/1
  Bus Selector/1 -> [turnOK]  "<wc_flag>"
  Bus Selector1/1 -> [vertOK]  "<wc_flag>"
  Relational Operator/1 -> MATLAB Function/1(preferTurn)  "true if prefer turn"
  MATLAB Function/1(chooseTurn) -> Scope/1, Switch1/2, Switch/2  "true if  turn"
  [vertOK] -> MATLAB Function/3(vert_flag)
  [turnOK] -> MATLAB Function/2(turn_flag)
  Switch/1 -> Unit Delay1/1, Bus Selector2/1, Hrz Maneuver/1
  Constant/1 -> Memory/1
  Memory/1 -> Switch2/2, Switch3/2
  Switch2/1 -> Switch/3
  Null Maneuver/1(Null) -> Switch2/1, Switch3/1
  Switch3/1 -> Switch1/1
  Unit Delay/1 -> Switch3/3
  Unit Delay1/1 -> Switch2/3
  Bus Selector2/1 -> Scope1/1  "<type>"
  Switch1/1 -> Unit Delay/1, Bus Selector3/1, Vrt Maneuver/1
  Bus Selector3/1 -> Scope2/1  "<type>"
  Constant2/1 -> Selector/1
  Abs/1 -> 1-D Lookup Table1/1
  Abs1/1 -> 1-D Lookup Table/1
  1-D Lookup Table1/1 -> Selector/2
  1-D Lookup Table/1 -> Selector/3
  Selector/1 -> Relational Operator/2
  Max Turn Rt/1 -> Abs1/1
  Max Vert Rt/1 -> Abs/1

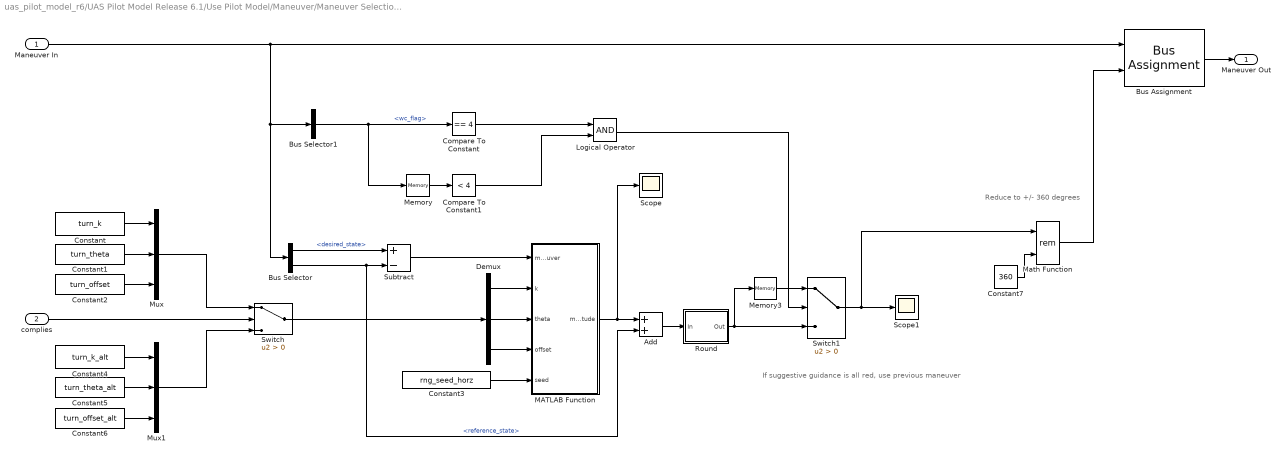
== system uas_pilot_model_r6/UAS Pilot Model Release 6.1/Use Pilot Model/Maneuver/Maneuver Selection/Draw Horizontal Magnitude ==
  note: Reduce to +/- 360 degrees
  note: If suggestive guidance is all red, use previous maneuver
  Maneuver In : Inport
  complies : Inport  Port=2
  Add : Sum
  Bus Assignment : BusAssignment  AssignedSignals=desired_state
  Bus Selector : BusSelector  OutputSignals=desired_state,reference_state
  Bus Selector1 : BusSelector  OutputSignals=wc_flag
  Compare To Constant : simulink/Logic and Bit Operations/Compare To Constant  relop===  const=4  OutDataTypeStr=boolean
  Compare To Constant1 : simulink/Logic and Bit Operations/Compare To Constant  relop=<  const=4  OutDataTypeStr=boolean
  Constant : Constant  Value=turn_k
  Constant1 : Constant  Value=turn_theta
  Constant2 : Constant  Value=turn_offset
  Constant3 : Constant  Value=rng_seed_horz
  Constant4 : Constant  Value=turn_k_alt
  Constant5 : Constant  Value=turn_theta_alt
  Constant6 : Constant  Value=turn_offset_alt
  Constant7 : Constant  Value=360
  Demux : Demux  Outputs=3
  Logical Operator : Logic  AllPortsSameDT=off  OutDataTypeStr=boolean
  MATLAB Function : MATLAB Function  TreatAsAtomicUnit=on
  Math Function : Math  Operator=rem  SaturateOnIntegerOverflow=on
  Memory : Memory  InitialCondition=4  InheritSampleTime=on
  Memory3 : Memory  InheritSampleTime=on
  Mux : Mux  Inputs=3
  Mux1 : Mux  Inputs=3
  Round : Subsystem  mask{factor=5}
      mask prompts: factor "Round to nearest:"
  Scope : Scope
  Scope1 : Scope
  Subtract : Sum  Inputs=+-
  Switch : Switch  Criteria=u2 > Threshold
  Switch1 : Switch  Criteria=u2 > Threshold
  Maneuver Out : Outport
  wires:
  Memory3/1 -> Switch1/1
  Compare To Constant/1 -> Logical Operator/1
  Maneuver In/1 -> Bus Assignment/1, Bus Selector1/1, Bus Selector/1
  Logical Operator/1 -> Switch1/2
  Compare To Constant1/1 -> Logical Operator/2
  Memory/1 -> Compare To Constant1/1
  Switch1/1 -> Math Function/1, Scope1/1
  Bus Selector1/1 -> Compare To Constant/1, Memory/1  "<wc_flag>"
  Switch/1 -> Demux/1
  complies/1 -> Switch/2
  Mux/1 -> Switch/1
  Mux1/1 -> Switch/3
  Constant6/1 -> Mux1/3
  Constant5/1 -> Mux1/2
  Constant4/1 -> Mux1/1
  Constant2/1 -> Mux/3
  Constant1/1 -> Mux/2
  Constant/1 -> Mux/1
  Round/1(Out) -> Switch1/3, Memory3/1
  Bus Selector/1 -> Subtract/1  "<desired_state>"
  Bus Selector/2 -> Add/2, Subtract/2  "<reference_state>"
  Subtract/1 -> MATLAB Function/1(maneuver)
  Demux/1 -> MATLAB Function/2(k)
  Demux/2 -> MATLAB Function/3(theta)
  Demux/3 -> MATLAB Function/4(offset)
  Constant3/1 -> MATLAB Function/5(seed)
  MATLAB Function/1(magnitude) -> Scope/1, Add/1
  Add/1 -> Round/1(In)
  Bus Assignment/1 -> Maneuver Out/1
  Math Function/1 -> Bus Assignment/2
  Constant7/1 -> Math Function/2

== system uas_pilot_model_r6/UAS Pilot Model Release 6.1/Use Pilot Model/Maneuver/Maneuver Selection/Draw Vertical Magnitude ==
  Own Vertical Direction : Inport
  Maneuver In : Inport  Port=2
  Altitude Floor : Subsystem  mask{alt_floor=500}
      mask prompts: alt_floor "Altitude Floor (feet)"
  Bus Assignment : BusAssignment  AssignedSignals=desired_state
  Bus Selector : BusSelector  OutputSignals=desired_state,reference_state
  Constant : Constant  Value=alt_k
  Constant1 : Constant  Value=alt_theta
  Constant2 : Constant  Value=alt_offset
  Constant3 : Constant  Value=rng_seed_vert
  MATLAB Function : MATLAB Function  TreatAsAtomicUnit=on
  Round Altitude : Subsystem
  Subtract : Sum  Inputs=+-
  Maneuver Out : Outport
  wires:
  Bus Assignment/1 -> Maneuver Out/1
  Maneuver In/1 -> Bus Assignment/1, Bus Selector/1
  Bus Selector/1 -> Subtract/1  "<desired_state>"
  Bus Selector/2 -> Altitude Floor/2(Reference Alt), Round Altitude/2(Reference Alt), Subtract/2  "<reference_state>"
  Subtract/1 -> MATLAB Function/1(maneuver)  "minimum maneuver"
  Constant/1 -> MATLAB Function/2(k)
  Constant1/1 -> MATLAB Function/3(theta)
  Constant2/1 -> MATLAB Function/4(offset)
  Constant3/1 -> MATLAB Function/5(seed)
  Altitude Floor/1(Alt Out) -> Bus Assignment/2
  MATLAB Function/1(magnitude) -> Round Altitude/1(Alt In)
  Round Altitude/1(Alt Out) -> Altitude Floor/1(Alt In)
  Own Vertical Direction/1 -> Round Altitude/3(Ownship Climb/Descend)

== system uas_pilot_model_r6/UAS Pilot Model Release 6.1/Use Pilot Model/Maneuver/Maneuver Selection/Get Minimum Maneuvers ==
  Own State : Inport
  Guidance : Inport  Port=2
  Bus Selector : BusSelector  OutputSignals=h_ft
  Get Minimum Altitudes : MATLAB Function  TreatAsAtomicUnit=on
  Get Minimum Turns : MATLAB Function  TreatAsAtomicUnit=on
  To Workspace : ToWorkspace  VariableName=minTurns  SaveFormat=Timeseries  SampleTime=-1
  To Workspace1 : ToWorkspace  VariableName=turnFlags  SaveFormat=Timeseries  SampleTime=-1
  To Workspace2 : ToWorkspace  VariableName=minAlt  SaveFormat=Timeseries  SampleTime=-1
  To Workspace3 : ToWorkspace  VariableName=altFlags  SaveFormat=Timeseries  SampleTime=-1
  turns : Outport
  turn flags : Outport  Port=2
  alts : Outport  Port=3
  alt flags : Outport  Port=4
  wires:
  Bus Selector/1 -> Get Minimum Altitudes/2(currAlt)  "<h_ft>"
  Own State/1 -> Bus Selector/1
  Guidance/1 -> Get Minimum Altitudes/1(bands), Get Minimum Turns/1(bands)
  Get Minimum Turns/1(turns) -> To Workspace/1, turns/1
  Get Minimum Turns/2(wc_flag) -> To Workspace1/1, turn flags/1
  Get Minimum Altitudes/1(alts) -> To Workspace2/1, alts/1
  Get Minimum Altitudes/2(wc_flag) -> To Workspace3/1, alt flags/1

== system uas_pilot_model_r6/UAS Pilot Model Release 6.1/Use Pilot Model/Maneuver/Maneuver Selection/Subsystem ==
  Alt Guidance : Inport
  Prev Maneuver : Inport  Port=2
  Bus Selector : BusSelector  OutputSignals=desired_state
  Bus Selector1 : BusSelector  OutputSignals=type
  Compare To Zero : simulink/Logic and Bit Operations/Compare To Zero  relop=>  OutDataTypeStr=boolean
  Demux : Demux  Outputs=2
  Logical Operator : Logic  Operator=OR  AllPortsSameDT=off  OutDataTypeStr=boolean
  Logical Operator1 : Logic  AllPortsSameDT=off  OutDataTypeStr=boolean
  Logical Operator2 : Logic  Operator=NOT  AllPortsSameDT=off  OutDataTypeStr=boolean
  Relational Operator : RelationalOperator  OutDataTypeStr=boolean  RndMeth=Nearest
  Relational Operator1 : RelationalOperator  OutDataTypeStr=boolean  RndMeth=Nearest
  Scope{,1..3} (4 alike) : Scope
  Re-draw : Outport
  wires:
  Logical Operator2/1 -> Re-draw/1, Scope/1
  Logical Operator1/1 -> Logical Operator2/1
  Logical Operator/1 -> Logical Operator1/2
  Compare To Zero/1 -> Logical Operator1/1
  Bus Selector1/1 -> Compare To Zero/1  "<type>"
  Relational Operator/1 -> Logical Operator/2
  Relational Operator1/1 -> Logical Operator/1
  Demux/2 -> Relational Operator/2, Scope3/1  "climb"
  Bus Selector/1 -> Relational Operator1/2, Relational Operator/1, Scope1/1  "<desired_state>"
  Demux/1 -> Relational Operator1/1, Scope2/1  "descend"
  Alt Guidance/1 -> Demux/1
  Prev Maneuver/1 -> Bus Selector/1, Bus Selector1/1

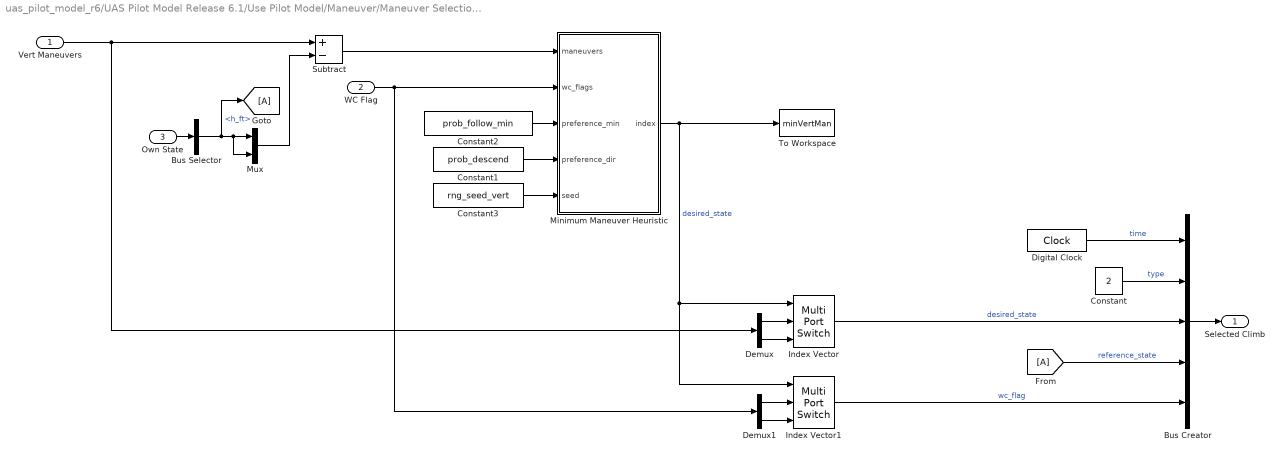
== system uas_pilot_model_r6/UAS Pilot Model Release 6.1/Use Pilot Model/Maneuver/Maneuver Selection/Vertical Maneuver Heuristic ==
  Vert Maneuvers : Inport
  WC Flag : Inport  Port=2
  Own State : Inport  Port=3
  Bus Selector : BusSelector  OutputSignals=h_ft
  Bus Creator : BusCreator  Inputs=5  OutDataTypeStr=Bus: AvoidanceManeuver
  Constant : Constant  Value=2
  Constant1 : Constant  Value=prob_descend
  Constant2 : Constant  Value=prob_follow_min
  Constant3 : Constant  Value=rng_seed_vert
  Demux : Demux  Outputs=2
  Demux1 : Demux  Outputs=2
  Digital Clock : DigitalClock  SampleTime=dt
  Index Vector : MultiPortSwitch  DataPortOrder=Specify indices  Inputs=1  DataPortIndices={1,2}
  Index Vector1 : MultiPortSwitch  DataPortOrder=Specify indices  Inputs=1  DataPortIndices={1,2}
  Minimum Maneuver Heuristic : MATLAB Function  TreatAsAtomicUnit=on
  Mux : Mux  Inputs=2
  Subtract : Sum  Inputs=+-
  To Workspace : ToWorkspace  VariableName=minVertMan  SaveFormat=Timeseries  SampleTime=-1
  Selected Climb : Outport
  wires:
  Index Vector/1 -> Bus Creator/3  "desired_state"
  Vert Maneuvers/1 -> Demux/1, Subtract/1
  Bus Creator/1 -> Selected Climb/1
  Digital Clock/1 -> Bus Creator/1  "time"
  Constant/1 -> Bus Creator/2  "type"
  Own State/1 -> Bus Selector/1
  Bus Selector/1 -> [A], Mux/2, Mux/1  "<h_ft>"
  [A] -> Bus Creator/4  "reference_state"
  Constant2/1 -> Minimum Maneuver Heuristic/3(preference_min)
  Constant3/1 -> Minimum Maneuver Heuristic/5(seed)
  Mux/1 -> Subtract/2
  Subtract/1 -> Minimum Maneuver Heuristic/1(maneuvers)
  WC Flag/1 -> Minimum Maneuver Heuristic/2(wc_flags), Demux1/1
  Index Vector1/1 -> Bus Creator/5  "wc_flag"
  Demux/2 -> Index Vector/3
  Demux/1 -> Index Vector/2
  Demux1/1 -> Index Vector1/2
  Demux1/2 -> Index Vector1/3
  Constant1/1 -> Minimum Maneuver Heuristic/4(preference_dir)
  Minimum Maneuver Heuristic/1(index) -> Index Vector/1, Index Vector1/1, To Workspace/1  "desired_state"

== system uas_pilot_model_r6/UAS Pilot Model Release 6.1/Use Pilot Model/Maneuver/Coordination Delay/Draw Coord Delay/Generate Random Gamma Deviate ==
  Add : Sum
  Constant : Constant  Value=offset
  MATLAB Function : MATLAB Function  TreatAsAtomicUnit=on
  Scale Parameter : Constant  Value=theta
  Seed : Constant  Value=seed
  Shape Parameter : Constant  Value=k
  y : Outport
  wires:
  Constant/1 -> Add/2
  Add/1 -> y/1
  Seed/1 -> MATLAB Function/3(seed)
  Scale Parameter/1 -> MATLAB Function/2(b)
  MATLAB Function/1(y) -> Add/1
  Shape Parameter/1 -> MATLAB Function/1(a)

== system uas_pilot_model_r6/UAS Pilot Model Release 6.1/Use Pilot Model/Maneuver/Initial Delay/Draw Initial Delay/Generate Random Exponential Deviate ==
  Add : Sum
  Constant : Constant  Value=offset
  MATLAB Function : MATLAB Function  TreatAsAtomicUnit=on
  Mean Parameter : Constant  Value=mu
  Seed : Constant  Value=seed
  y : Outport
  wires:
  Add/1 -> y/1
  Constant/1 -> Add/2
  Seed/1 -> MATLAB Function/2(seed)
  MATLAB Function/1(y) -> Add/1
  Mean Parameter/1 -> MATLAB Function/1(a)

== system uas_pilot_model_r6/UAS Pilot Model Release 6.1/Use Pilot Model/Maneuver/Maneuver Selection/Choose Maneuver/Null Maneuver ==
  Bus Creator : BusCreator  Inputs=5  OutDataTypeStr=Bus: AvoidanceManeuver
  Constant{,1..3} (4 alike) : Constant  Value=0
  Digital Clock : DigitalClock  SampleTime=dt
  Null : Outport
  wires:
  Constant2/1 -> Bus Creator/5  "wc_flag"
  Constant/1 -> Bus Creator/2  "type"
  Constant1/1 -> Bus Creator/3  "desired_state"
  Digital Clock/1 -> Bus Creator/1  "time"
  Bus Creator/1 -> Null/1
  Constant3/1 -> Bus Creator/4  "reference_state"

== system uas_pilot_model_r6/UAS Pilot Model Release 6.1/Use Pilot Model/Maneuver/Maneuver Selection/Draw Horizontal Magnitude/Round ==
  In : Inport
  Constant : Constant  Value=factor
  Divide : Product  Inputs=*/
  Product : Product
  Rounding Function : Rounding  Operator=round
  Out : Outport
  wires:
  Product/1 -> Out/1
  Constant/1 -> Divide/2, Product/2
  Divide/1 -> Rounding Function/1
  In/1 -> Divide/1
  Rounding Function/1 -> Product/1

== system uas_pilot_model_r6/UAS Pilot Model Release 6.1/Use Pilot Model/Maneuver/Maneuver Selection/Draw Vertical Magnitude/Altitude Floor ==
  note: If the reference altitude is > 500 ft, don't let the commanded
      | altitude be anything less than 500 ft.
  Alt In : Inport
  Reference Alt : Inport  Port=2
  Constant4 : Constant  Value=alt_floor
  MinMax : MinMax  Function=max  Inputs=2
  Relational Operator : RelationalOperator  Operator=<=  OutDataTypeStr=boolean  RndMeth=Nearest
  Switch : Switch  Criteria=u2 > Threshold
  Alt Out : Outport
  wires:
  Relational Operator/1 -> Switch/2
  Constant4/1 -> Relational Operator/2, MinMax/2
  Alt In/1 -> MinMax/1, Switch/1
  MinMax/1 -> Switch/3
  Switch/1 -> Alt Out/1
  Reference Alt/1 -> Relational Operator/1

== system uas_pilot_model_r6/UAS Pilot Model Release 6.1/Use Pilot Model/Maneuver/Maneuver Selection/Draw Vertical Magnitude/Round Altitude ==
  note: Round to nearest 100 ft unless desired alt == reference alt and ownship is level
  Alt In : Inport
  Reference Alt : Inport  Port=2
  Ownship Climb/Descend : Inport  Port=3
  Add : Sum
  Compare To Zero : simulink/Logic and Bit Operations/Compare To Zero  relop=~=  OutDataTypeStr=boolean
  Compare To Zero1 : simulink/Logic and Bit Operations/Compare To Zero  relop=~=  OutDataTypeStr=boolean
  Logical Operator : Logic  Operator=OR  AllPortsSameDT=off  OutDataTypeStr=boolean
  Round : Subsystem  mask{factor=100}
      mask prompts: factor "Round to nearest:"
  Scope : Scope
  Scope1 : Scope
  Scope2 : Scope
  Switch1 : Switch  Criteria=u2 > Threshold
  Alt Out : Outport
  wires:
  Alt In/1 -> Add/1, Compare To Zero/1
  Add/1 -> Scope2/1, Switch1/3, Round/1(In)
  Round/1(Out) -> Switch1/1
  Reference Alt/1 -> Add/2
  Switch1/1 -> Alt Out/1
  Ownship Climb/Descend/1 -> Compare To Zero1/1
  Logical Operator/1 -> Switch1/2
  Compare To Zero/1 -> Scope1/1, Logical Operator/2
  Compare To Zero1/1 -> Logical Operator/1, Scope/1

== system uas_pilot_model_r6/UAS Pilot Model Release 6.1/Use Pilot Model/Maneuver/Maneuver Selection/Draw Vertical Magnitude/Round Altitude/Round ==
  In : Inport
  Constant : Constant  Value=factor
  Divide : Product  Inputs=*/
  Product : Product
  Rounding Function : Rounding  Operator=round
  Out : Outport
  wires:
  Product/1 -> Out/1
  Constant/1 -> Divide/2, Product/2
  Divide/1 -> Rounding Function/1
  In/1 -> Divide/1
  Rounding Function/1 -> Product/1

== matlab function uas_pilot_model_r6/UAS Pilot Model Release 6.1/Use Pilot Model/Maneuver/Coordination Delay/Draw Coord Delay/Generate Random Gamma Deviate/MATLAB Function ==
  data: a input; y output; b input; seed input
function y = fcn(a, b, seed)
%#codegen

info = rng;
if info.Seed ~= seed
  rng(seed);
end

y = HeuristicOperatorModelR6_ExternalFunctions.gammaDeviate(a,b);

== matlab function uas_pilot_model_r6/UAS Pilot Model Release 6.1/Use Pilot Model/Maneuver/Initial Delay/Draw Initial Delay/Generate Random Exponential Deviate/MATLAB Function ==
  data: a input; y output; seed input
function y = fcn(a, seed)
%#codegen

info = rng;
if info.Seed ~= seed
  rng(seed);
end

y = HeuristicOperatorModelR6_ExternalFunctions.exponentialDeviate(a);

== matlab function uas_pilot_model_r6/UAS Pilot Model Release 6.1/Use Pilot Model/Maneuver/Maneuver Selection/Choose Horizontal Maneuver/Minimum Maneuver Heuristic ==
  data: maneuvers input; index output; wc_flags input; preference_min input; preference_dir input; max_diff input; seed input; isMin output
function [index, isMin] = fcn(maneuvers, wc_flags, preference_min, preference_dir, max_diff, seed)
%#codegen

index = 0;
isMin = true;
[index, isMin] = HeuristicOperatorModelR6_ExternalFunctions.chooseMinimumManeuver(maneuvers, wc_flags, preference_min, preference_dir, max_diff, seed);

== matlab function uas_pilot_model_r6/UAS Pilot Model Release 6.1/Use Pilot Model/Maneuver/Maneuver Selection/Choose Maneuver/MATLAB Function ==
  data: preferTurn input; chooseTurn output; turn_flag input; vert_flag input
function chooseTurn = fcn(preferTurn, turn_flag, vert_flag)
%#codegen

chooseTurn = 1; %#ok<NASGU>
chooseTurn = HeuristicOperatorModelR6_ExternalFunctions.chooseBetweenHorzAndVert(preferTurn, turn_flag, vert_flag);

== matlab function uas_pilot_model_r6/UAS Pilot Model Release 6.1/Use Pilot Model/Maneuver/Maneuver Selection/Draw Horizontal Magnitude/MATLAB Function ==
  data: maneuver input; magnitude output; k input; theta input; offset input; seed input
function magnitude = fcn(maneuver, k, theta, offset, seed)
%#codegen

magnitude = HeuristicOperatorModelR6_ExternalFunctions.drawManeuverMagnitude(maneuver, k, theta, offset, seed);
